simulink model "Simulation_6Pulse_IGBT_Three_Phase"  (R2024b)
settings: Solver=FixedStepAuto  StartTime=0.0  StopTime=0.002  FixedStep=1e-6  RelTol=1e-3  EnableMultiTasking=on
libraries: c2837xDlib x6, spsIGBTDiodeLib x6, spsVoltageMeasurementLib x3, spsDCVoltageSourceLib x1, c2000lib x1, spsGroundLib x1, dspstat3 x1, simulink x1, spsThreePhaseSeriesRLCBranchLib x1, spsThreePhaseVIMeasurementLib x1, sps_lib x1
settings Model: ExtModeTrigDuration=8  Creator=sina  LastModifiedBy=sina
settings OptimizationCC: DefaultParameterBehavior=Inlined  DefaultUnderspecifiedDataType=single  EnhancedBackFolding=on  PassReuseOutputArgsAs=Individual arguments  MaxStackSize=1024  OptimizeBlockOrder=speed  DifferentSizesBufferReuse=on  OptimizationCustomize=off  EfficientTunableParamExpr=on
settings DebuggingCC: ParameterTunabilityLossMsg=error
settings HardwareCC: ProdBitPerChar=16  ProdBitPerInt=16  ProdBitPerPointer=32  ProdBitPerSizeT=32  ProdBitPerPtrDiffT=32  ProdLargestAtomicInteger=Integer  ProdLargestAtomicFloat=None  ProdWordSize=16  ProdLongLongMode=on  ProdHWDeviceType=Texas Instruments->C2000  HardwareBoardFeatureSet=SoCBlockset
settings SFSimCC: MATLABDynamicMemAlloc=off
settings RTWCC: Description=Embedded Coder  SystemTargetFile=ert.tlc  HardwareBoard=TI Delfino F2837xD  TemplateMakefile=ert_default_tmf  Toolchain=Texas Instruments Code Composer Studio (C2000)  CodeProfilingSaveOptions=MetricsOnly
settings CodeAppCC: ForceParamTrailComments=on  IgnoreCustomStorageClasses=off  OperatorAnnotations=on  SimulinkDataObjDesc=on  SFDataObjDesc=on  InsertBlockDesc=on
settings ERTTargetCC: CodeReplacementLibrary=TI C28x,TI C28x with C99 extensions  SupportContinuousTime=on  ExtModeTransport=4  ExtModeStaticAlloc=on  ExtModeAutomaticAllocSize=off  ExtModeStaticAllocSize=10000  ExtModeMexFile=ext_xcp  ExtModeIntrfLevel=Level2 - Open

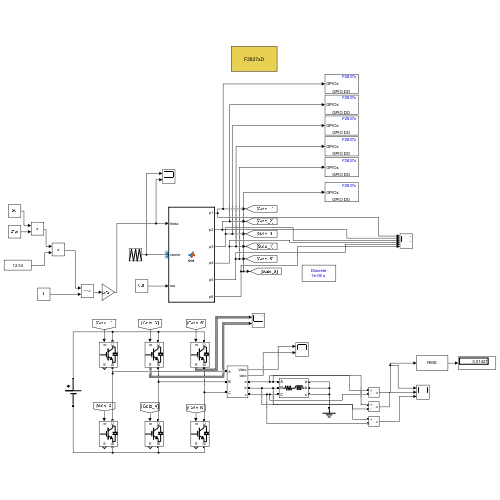
[thumbnail: Simulink's stored preview of the top-level diagram]
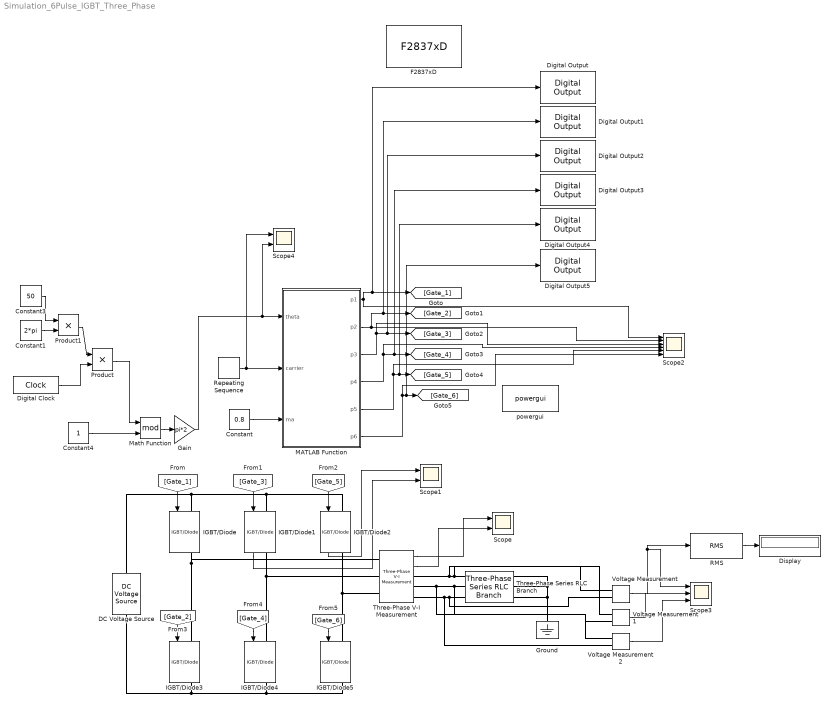
== system Simulation_6Pulse_IGBT_Three_Phase ==
  Constant : Constant  Value=0.8
  Constant1 : Constant  Value=2*pi
  Constant3 : Constant  Value=50
  Constant4 : Constant
  DC Voltage Source : spsDCVoltageSourceLib/DC Voltage Source  Amplitude=100  Measurements=None
  Digital Clock : DigitalClock  SampleTime=1e-6
  Digital Output : c2837xDlib/Digital Output  GPIO_Number=GPIO0~GPIO7  GPIO_Bit0=on  GPIO_BIT0_Toggle=off  GPIO_Bit1=off  GPIO_BIT1_Toggle=off  GPIO_Bit2=off  GPIO_BIT2_Toggle=off  GPIO_Bit3=off  GPIO_BIT3_Toggle=off  GPIO_Bit4=off  GPIO_BIT4_Toggle=off  GPIO_Bit5=off  GPIO_BIT5_Toggle=off  GPIO_Bit6=off  GPIO_BIT6_Toggle=off  GPIO_Bit7=off  GPIO_BIT7_Toggle=off
  Digital Output1 : c2837xDlib/Digital Output  GPIO_Number=GPIO0~GPIO7  GPIO_Bit0=off  GPIO_BIT0_Toggle=off  GPIO_Bit1=on  GPIO_BIT1_Toggle=off  GPIO_Bit2=off  GPIO_BIT2_Toggle=off  GPIO_Bit3=off  GPIO_BIT3_Toggle=off  GPIO_Bit4=off  GPIO_BIT4_Toggle=off  GPIO_Bit5=off  GPIO_BIT5_Toggle=off  GPIO_Bit6=off  GPIO_BIT6_Toggle=off  GPIO_Bit7=off  GPIO_BIT7_Toggle=off
  Digital Output2 : c2837xDlib/Digital Output  GPIO_Number=GPIO0~GPIO7  GPIO_Bit0=off  GPIO_BIT0_Toggle=off  GPIO_Bit1=off  GPIO_BIT1_Toggle=off  GPIO_Bit2=on  GPIO_BIT2_Toggle=off  GPIO_Bit3=off  GPIO_BIT3_Toggle=off  GPIO_Bit4=off  GPIO_BIT4_Toggle=off  GPIO_Bit5=off  GPIO_BIT5_Toggle=off  GPIO_Bit6=off  GPIO_BIT6_Toggle=off  GPIO_Bit7=off  GPIO_BIT7_Toggle=off
  Digital Output3 : c2837xDlib/Digital Output  GPIO_Number=GPIO0~GPIO7  GPIO_Bit0=off  GPIO_BIT0_Toggle=off  GPIO_Bit1=off  GPIO_BIT1_Toggle=off  GPIO_Bit2=off  GPIO_BIT2_Toggle=off  GPIO_Bit3=on  GPIO_BIT3_Toggle=off  GPIO_Bit4=off  GPIO_BIT4_Toggle=off  GPIO_Bit5=off  GPIO_BIT5_Toggle=off  GPIO_Bit6=off  GPIO_BIT6_Toggle=off  GPIO_Bit7=off  GPIO_BIT7_Toggle=off
  Digital Output4 : c2837xDlib/Digital Output  GPIO_Number=GPIO0~GPIO7  GPIO_Bit0=off  GPIO_BIT0_Toggle=off  GPIO_Bit1=off  GPIO_BIT1_Toggle=off  GPIO_Bit2=off  GPIO_BIT2_Toggle=off  GPIO_Bit3=off  GPIO_BIT3_Toggle=off  GPIO_Bit4=on  GPIO_BIT4_Toggle=off  GPIO_Bit5=off  GPIO_BIT5_Toggle=off  GPIO_Bit6=off  GPIO_BIT6_Toggle=off  GPIO_Bit7=off  GPIO_BIT7_Toggle=off
  Digital Output5 : c2837xDlib/Digital Output  GPIO_Number=GPIO0~GPIO7  GPIO_Bit0=off  GPIO_BIT0_Toggle=off  GPIO_Bit1=off  GPIO_BIT1_Toggle=off  GPIO_Bit2=off  GPIO_BIT2_Toggle=off  GPIO_Bit3=off  GPIO_BIT3_Toggle=off  GPIO_Bit4=off  GPIO_BIT4_Toggle=off  GPIO_Bit5=on  GPIO_BIT5_Toggle=off  GPIO_Bit6=off  GPIO_BIT6_Toggle=off  GPIO_Bit7=off  GPIO_BIT7_Toggle=off
  Display : Display
  F2837xD : c2000lib/F2837xD  SystemSampleTime=-1  VariantActivationTime=update diagram  AllowFlexibleInterface=on  Latency=0  AutoFrameSizeCalculation=off
  Gain : Gain  Gain=pi*2
  Ground : spsGroundLib/Ground  LConnTagsString=a
  IGBT/Diode{,1..5} (6 alike) : spsIGBTDiodeLib/IGBT//Diode  Ron=1e-3  Rs=1e5  Cs=inf  Measurements=on
  MATLAB Function : MATLAB Function  TreatAsAtomicUnit=on
  Math Function : Math  Operator=mod
  Product : Product
  Product1 : Product
  RMS : dspstat3/RMS  run=off  directionMode=Each column  dimension=1  InputProcessing=Columns as channels (frame based)  reset_popup=None
  Repeating Sequence : simulink/Sources/Repeating Sequence  rep_seq_t=[0 0.000025 0.00005]  rep_seq_y=[-1 1 -1]
  Scope : Scope  NumInputPorts=2
  Scope1 : Scope  NumInputPorts=2
  Scope2 : Scope  NumInputPorts=6
  Scope3 : Scope  NumInputPorts=3
  Scope4 : Scope  NumInputPorts=2
  Three-Phase Series RLC Branch : spsThreePhaseSeriesRLCBranchLib/Three-Phase Series RLC Branch  LConnTagsString=A|B|C  RConnTagsString=A|B|C  BranchType=RL  Resistance=1  Inductance=3e-3  Capacitance=1e-6  Measurements=None
  Three-Phase V-I Measurement : spsThreePhaseVIMeasurementLib/Three-Phase V-I Measurement  VoltageMeasurement=phase-to-phase  SetLabelV=off  LabelV=Vabc  Vpu=off  VpuLL=off  CurrentMeasurement=yes  SetLabelI=off  LabelI=Iabc  Ipu=off  Pbase=100e6  Vbase=500e3  OutputType=Complex  PhasorSimulation=off  PSBequivalent=0
  Voltage Measurement : spsVoltageMeasurementLib/Voltage Measurement  PhasorSimulation=off  OutputType=Complex  PSBequivalent=0
  Voltage Measurement1 : spsVoltageMeasurementLib/Voltage Measurement  PhasorSimulation=off  OutputType=Complex  PSBequivalent=0
  Voltage Measurement2 : spsVoltageMeasurementLib/Voltage Measurement  PhasorSimulation=off  OutputType=Complex  PSBequivalent=0
  powergui : sps_lib/powergui  Priority=1  SimulationMode=Discrete  SampleTime=1e-6  frequency=60  Iterations=50  frequencyindice=0  Pbase=100e6  ErrMax=1e-4  UnitsV=kV  UnitsW=MW  buscounter=0  FunctionMessages=off  echomessages=off  EnableUseOfTLC=off  CurrentSourceSwitches=off  DisableSnubberDevices=off  DisableRonSwitches=off  DisableVfSwitches=off  DisplayEquations=off  AutomaticDiscreteSolvers=off  SolverType=Tustin/Backward Euler (TBE)  Interpol=off  ExternalGateDelay=off  methode=off  Ts=100  x0status=blocks  SPID=on  SwTol=0  HookPort=off  NonlinearTolerance=1e-4  nMaxIteration=100  ContinueOnMaxIteration=off  RestoreLinks=warning  ResistiveCurrentMeasurement=off  Frange=[0:2:500]  Ylog=off  Xlog=on  ShowGrid=off  save=off  variable=ZData  structure=0  ZoomFFT=off  StartTime=0.0  cycles=1  DisplayStyle=1  fundamental=60  FreqAxis=off  MaxFrequency=1000  frequencyindicesteady=1  RmsSteady=1  display=off
  wires:
  MATLAB Function/1(p1) -> [Gate_1], Digital Output/1, Scope2/1
  MATLAB Function/2(p2) -> Digital Output1/1, [Gate_2], Scope2/2
  MATLAB Function/3(p3) -> Digital Output2/1, [Gate_3], Scope2/3
  MATLAB Function/4(p4) -> Digital Output3/1, [Gate_4], Scope2/4
  MATLAB Function/5(p5) -> Scope2/5, Digital Output4/1, [Gate_5]
  MATLAB Function/6(p6) -> Scope2/6, Digital Output5/1, [Gate_6]
  [Gate_1] -> IGBT/Diode/1
  [Gate_3] -> IGBT/Diode1/1
  [Gate_5] -> IGBT/Diode2/1
  [Gate_2] -> IGBT/Diode3/1
  [Gate_4] -> IGBT/Diode4/1
  [Gate_6] -> IGBT/Diode5/1
  Constant/1 -> MATLAB Function/3(ma)
  Repeating Sequence/1 -> Scope4/1, MATLAB Function/2(carrier)
  Three-Phase V-I Measurement/1 -> Scope/1
  IGBT/Diode2/1 -> Scope1/1
  IGBT/Diode1/1 -> Scope1/2
  Three-Phase V-I Measurement/2 -> Scope/2
  Digital Clock/1 -> Product/2
  Constant4/1 -> Math Function/2
  Product/1 -> Math Function/1
  Math Function/1 -> Gain/1
  Gain/1 -> Scope4/2, MATLAB Function/1(theta)
  Voltage Measurement/1 -> RMS/1, Scope3/1
  RMS/1 -> Display/1
  Voltage Measurement1/1 -> Scope3/2
  Voltage Measurement2/1 -> Scope3/3
  Product1/1 -> Product/1
  Constant3/1 -> Product1/1
  Constant1/1 -> Product1/2
  connections:
  IGBT/Diode/LConn1 -- IGBT/Diode2/LConn1 -- IGBT/Diode1/LConn1 -- DC Voltage Source/RConn1
  IGBT/Diode1/RConn1 -- Three-Phase V-I Measurement/LConn2 -- IGBT/Diode4/LConn1
  IGBT/Diode2/RConn1 -- Three-Phase V-I Measurement/LConn3 -- IGBT/Diode5/LConn1
  IGBT/Diode/RConn1 -- Three-Phase V-I Measurement/LConn1 -- IGBT/Diode3/LConn1
  IGBT/Diode5/RConn1 -- IGBT/Diode4/RConn1 -- DC Voltage Source/LConn1 -- IGBT/Diode3/RConn1
  Three-Phase V-I Measurement/RConn1 -- Voltage Measurement1/LConn1 -- Three-Phase Series RLC Branch/LConn1 -- Voltage Measurement/LConn1
  Three-Phase Series RLC Branch/LConn2 -- Voltage Measurement1/LConn2 -- Voltage Measurement2/LConn1 -- Three-Phase V-I Measurement/RConn2
  Three-Phase Series RLC Branch/LConn3 -- Voltage Measurement/LConn2 -- Voltage Measurement2/LConn2 -- Three-Phase V-I Measurement/RConn3
  Ground/LConn1 -- Three-Phase Series RLC Branch/RConn3 -- Three-Phase Series RLC Branch/RConn2 -- Three-Phase Series RLC Branch/RConn1

== matlab function Simulation_6Pulse_IGBT_Three_Phase/MATLAB Function ==
  data: theta input; carrier input; ma input; p1 output; p2 output; p3 output; p4 output; p5 output; p6 output
function [p1, p2, p3, p4, p5, p6] = fcn(theta, carrier, ma)
    % Set Dead-time value (typically between 0 and 0.1)
    % A larger value increases the blanking time between complementary switches
    dt = 0.05; 

    % 1. Generate reference sinusoidal modulating waves
    Va = ma * sin(theta);
    Vb = ma * sin(theta - 2*pi/3);
    Vc = ma * sin(theta + 2*pi/3);

    % 2. Generate gate pulses with Dead-time insertion
    % Upper switch turns ON when the sine wave exceeds (Carrier + dt)
    p1 = double( Va > (carrier + dt) );
    % Lower switch turns ON when the sine wave is below (Carrier - dt)
    p2 = double( Va < (carrier - dt) );

    % Phase B Gate Signals
    p3 = double( Vb > (carrier + dt) );
    p4 = double( Vb < (carrier - dt) );

    % Phase C Gate Signals
    p5 = double( Vc > (carrier + dt) );
    p6 = double( Vc < (carrier - dt) );
end
